simulink library "tpm"  (R2021b)
settings: Solver=VariableStepAuto  StartTime=0.0  StopTime=10.0  RelTol=1e-3
undefined symbols (not defined in the file or in its folder): ENUM_AN_LF, ENUM_AN_LR, ENUM_AN_RF, ENUM_AN_RR, ENUM_POWERSTA_OFF, ENUM_POWERSTA_OFFA, ENUM_POWERSTA_OFFC, ENUM_POWERSTA_ON, ENUM_POWERSTA_READY, ENUM_POWERSTA_STANDBY, ENUM_PWRSTASW_OFF, ENUM_PWRSTASW_OFFA, ENUM_PWRSTASW_OFFCHVCHRG, ENUM_PWRSTASW_STANDBY, KTPM_Delay_raw8, KTPM_WhlRotDir_enum_ovrdflg, KTPM_WhlRotDir_enum_ovrdval, TRUE, ZERO_FLOAT, ZERO_INT
libraries: simulink x58, hcu_lib x25, $bdroot x18
(part 6 of 8)

== system tpm/TPM/TPMS/TPMS/Learn/AutoLocation/IDIdentify/unlearnsensorfail  ==
  VTPM_ALLFIN_flg : Inport
  VINP_VehSpeed_kph : Inport  Port=2
  VTPM_IDLOCK_flg : Inport  Port=3
  GS1 : Inport  Port=4
  GS2 : Inport  Port=5
  GS3 : Inport  Port=6
  GS4 : Inport  Port=7
  VINP_TPMSResButt_flg : Inport  Port=8
  VINP_FlashunlearnSfali_flg : Inport  Port=9
  VINP_ChkStorge_flg : Inport  Port=10
  VINP_TPMSStorge_flg : Inport  Port=11
  Chart : Stateflow chart  TreatAsAtomicUnit=on
      settings: PortSchema="{\"entries\":[{\"content\":{\"sides\":[{\"content\":{\"connectorIds\":[\"In1\",\"In2\",\"In3\",\"In7\",\"In4\",\"In5\",\"In6\",\"In8\",\"In9\",\"In10\",\"In11\"]},\"type\":\"ConnectorPlacement.EquallySpacedRectSide\",\"uuid\":\"6d6ad79b-53cb-4fcc-b2ed-afc1b708014e\"},{\"content\":{\"connectorIds\":[\"Out1\",\"Out2\"],\"side\":\"RIGHT\"},\"type\":\"ConnectorPlacement.EquallySpacedRectSide\",\"uuid\":\"e1142f2b-ba58-4cb3-ba57-f7dfdeb40e8a\"},{\"content\":{\"connectorIds\":[],\"side\":\"TOP\"},\"type\":\"ConnectorPlacement.EquallySpacedRectSide\",\"uuid\":\"d6c2cba7-0cc1-4e16-8027-e1abdfd1a8ea\"}]},\"type\":\"ConnectorPlacement.EquallySpacedConnector\",\"uuid\":\"635c654b-7cdc-40ae-8580-2307d04d13e7\"}],\"packageUris\":[\"http://schema.mathworks.com/mf0/Connector/R2020b\"],\"version\":\"1.0\"}"
  Detect Increase4 : simulink/Logic and Bit Operations/Detect Increase  vinit=0.0  OutDataTypeStr=boolean
  SR_Latch : hcu_lib/Basic_Blocks/SR_Latch
  VTPM_unlearnSfali_flg : Outport
  VTPM_unlearnSfailvalid_enum : Outport  Port=2
  VTPM_unlockpopup_flg : Outport  Port=3
  wires:
  Chart/1(VTPM_unlearnSfali_flg) -> VTPM_unlearnSfali_flg/1, [VTPM_unlearnSfali_flg]
  GS1/1 -> Chart/7(VTPM_GS1_flg)
  GS4/1 -> Chart/6(VTPM_GS4_flg)
  GS3/1 -> Chart/5(VTPM_GS3_flg)
  GS2/1 -> Chart/4(VTPM_GS2_flg)
  VTPM_IDLOCK_flg/1 -> Chart/3(VTPM_IDLOCK_flg)
  VINP_VehSpeed_kph/1 -> Chart/2(VINP_VehSpeed_kph)
  VTPM_ALLFIN_flg/1 -> Chart/1(VTPM_ALLFIN_flg)
  VINP_FlashunlearnSfali_flg/1 -> Chart/9(VINP_FlashunlearnSfali_flg)
  VINP_ChkStorge_flg/1 -> Chart/10(VINP_ChkStorge_flg)
  VINP_TPMSStorge_flg/1 -> Chart/11(VINP_TPMSStorge_flg)
  SR_Latch/1 -> VTPM_unlearnSfailvalid_enum/1
  Detect Increase4/1 -> SR_Latch/1
  [VTPM_unlearnSfali_flg] -> Detect Increase4/1
  VINP_TPMSResButt_flg/1 -> [VINP_TPMSResButt_flg]
  [VINP_TPMSResButt_flg] -> Chart/8(VINP_TPMSResButt_flg)
  [VINP_TPMSResButt_flg] -> SR_Latch/2
  Chart/2(VTPM_unlockpopup_flg) -> VTPM_unlockpopup_flg/1

== system tpm/TPM/TPMS/TPMS/Learn/AutoLocation/WheelPosition/Subsystem ==
  VTPM_LFWpos_raw : Inport
  Constant : Constant  Value=KTPM_Delay_raw8
  If : If  IfExpression=u1 == 1  ElseIfExpressions=u1 ==2,u1 ==3,u1 ==4,u1 == 5,u1 ==6,u1 ==7,u1 ==8
  Merge1 : Merge  Inputs=9
  delay0 : Subsystem  TreatAsAtomicUnit=on
  delay1 : Subsystem  TreatAsAtomicUnit=on
  delay2 : Subsystem  TreatAsAtomicUnit=on
  delay3 : Subsystem  TreatAsAtomicUnit=on
  delay4 : Subsystem  TreatAsAtomicUnit=on
  delay5 : Subsystem  TreatAsAtomicUnit=on
  delay6 : Subsystem  TreatAsAtomicUnit=on
  delay7 : Subsystem  TreatAsAtomicUnit=on
  delay8 : Subsystem  TreatAsAtomicUnit=on
  VTPM_LFWP_raw16 : Outport
  wires:
  [VTPM_LFWP_raw16] -> delay3/1(In1)
  [VTPM_LFWP_raw16] -> delay1/1(In1)
  Constant/1 -> If/1
  Merge1/1 -> VTPM_LFWP_raw16/1
  [VTPM_LFWP_raw16] -> delay6/1(In1)
  [VTPM_LFWP_raw16] -> delay5/1(In1)
  [VTPM_LFWP_raw16] -> delay2/1(In1)
  [VTPM_LFWP_raw16] -> delay4/1(In1)
  [VTPM_LFWP_raw16] -> delay0/1(In1)
  VTPM_LFWpos_raw/1 -> [VTPM_LFWP_raw16]
  If/1 -> delay1/Action
  If/2 -> delay2/Action
  If/3 -> delay3/Action
  If/4 -> delay4/Action
  If/5 -> delay5/Action
  If/6 -> delay6/Action
  If/9 -> delay0/Action
  delay5/1(Out1) -> Merge1/5
  delay4/1(Out1) -> Merge1/4
  delay1/1(Out1) -> Merge1/1
  delay3/1(Out1) -> Merge1/3
  delay6/1(Out1) -> Merge1/6
  delay2/1(Out1) -> Merge1/2
  If/7 -> delay7/Action
  [VTPM_LFWP_raw16] -> delay7/1(In1)
  [VTPM_LFWP_raw16] -> delay8/1(In1)
  If/8 -> delay8/Action
  delay7/1(Out1) -> Merge1/7
  delay8/1(Out1) -> Merge1/8
  delay0/1(Out1) -> Merge1/9

== system tpm/TPM/TPMS/TPMS/Learn/AutoLocation/WheelPosition/Subsystem1 ==
  VTPM_RFWpos_raw : Inport
  Constant : Constant  Value=KTPM_Delay_raw8
  If : If  IfExpression=u1 == 1  ElseIfExpressions=u1 ==2,u1 ==3,u1 ==4,u1 == 5,u1 ==6,u1 ==7,u1 ==8
  Merge1 : Merge  Inputs=9
  delay0 : $bdroot/TPM/TPMS/TPMS/Learn/AutoLocation/WheelPosition/Subsystem/delay0  SystemSampleTime=-1  VariantActivationTime=update diagram  Latency=0  AutoFrameSizeCalculation=off
  delay1 : $bdroot/TPM/TPMS/TPMS/Learn/AutoLocation/WheelPosition/Subsystem/delay1  SystemSampleTime=-1  VariantActivationTime=update diagram  Latency=0  AutoFrameSizeCalculation=off
  delay2 : $bdroot/TPM/TPMS/TPMS/Learn/AutoLocation/WheelPosition/Subsystem/delay2  SystemSampleTime=-1  VariantActivationTime=update diagram  Latency=0  AutoFrameSizeCalculation=off
  delay3 : $bdroot/TPM/TPMS/TPMS/Learn/AutoLocation/WheelPosition/Subsystem/delay3  SystemSampleTime=-1  VariantActivationTime=update diagram  Latency=0  AutoFrameSizeCalculation=off
  delay4 : $bdroot/TPM/TPMS/TPMS/Learn/AutoLocation/WheelPosition/Subsystem/delay4  SystemSampleTime=-1  VariantActivationTime=update diagram  Latency=0  AutoFrameSizeCalculation=off
  delay5 : $bdroot/TPM/TPMS/TPMS/Learn/AutoLocation/WheelPosition/Subsystem/delay5  SystemSampleTime=-1  VariantActivationTime=update diagram  Latency=0  AutoFrameSizeCalculation=off
  delay6 : $bdroot/TPM/TPMS/TPMS/Learn/AutoLocation/WheelPosition/Subsystem/delay6  SystemSampleTime=-1  VariantActivationTime=update diagram  Latency=0  AutoFrameSizeCalculation=off
  delay7 : $bdroot/TPM/TPMS/TPMS/Learn/AutoLocation/WheelPosition/Subsystem/delay7  SystemSampleTime=-1  VariantActivationTime=update diagram  Latency=0  AutoFrameSizeCalculation=off
  delay8 : $bdroot/TPM/TPMS/TPMS/Learn/AutoLocation/WheelPosition/Subsystem/delay8  SystemSampleTime=-1  VariantActivationTime=update diagram  Latency=0  AutoFrameSizeCalculation=off
  VTPM_RFWP_raw16 : Outport
  wires:
  Merge1/1 -> VTPM_RFWP_raw16/1
  VTPM_RFWpos_raw/1 -> [VTPM_RFWP_raw16]
  [VTPM_RFWP_raw16] -> delay7/1
  delay7/1 -> Merge1/7
  delay8/1 -> Merge1/8
  delay0/1 -> Merge1/9
  [VTPM_RFWP_raw16] -> delay8/1
  [VTPM_RFWP_raw16] -> delay3/1
  If/2 -> delay2/Action
  [VTPM_RFWP_raw16] -> delay2/1
  [VTPM_RFWP_raw16] -> delay4/1
  If/1 -> delay1/Action
  [VTPM_RFWP_raw16] -> delay1/1
  If/9 -> delay0/Action
  If/3 -> delay3/Action
  [VTPM_RFWP_raw16] -> delay0/1
  delay2/1 -> Merge1/2
  delay5/1 -> Merge1/5
  [VTPM_RFWP_raw16] -> delay5/1
  delay6/1 -> Merge1/6
  If/6 -> delay6/Action
  If/8 -> delay8/Action
  delay3/1 -> Merge1/3
  If/5 -> delay5/Action
  [VTPM_RFWP_raw16] -> delay6/1
  If/4 -> delay4/Action
  delay4/1 -> Merge1/4
  delay1/1 -> Merge1/1
  If/7 -> delay7/Action
  Constant/1 -> If/1

== system tpm/TPM/TPMS/TPMS/Learn/AutoLocation/WheelPosition/Subsystem2 ==
  VTPM_LRWpos_raw : Inport
  Constant : Constant  Value=KTPM_Delay_raw8
  If : If  IfExpression=u1 == 1  ElseIfExpressions=u1 ==2,u1 ==3,u1 ==4,u1 == 5,u1 ==6,u1 ==7,u1 ==8
  Merge1 : Merge  Inputs=9
  delay0 : $bdroot/TPM/TPMS/TPMS/Learn/AutoLocation/WheelPosition/Subsystem/delay0  SystemSampleTime=-1  VariantActivationTime=update diagram  Latency=0  AutoFrameSizeCalculation=off
  delay1 : $bdroot/TPM/TPMS/TPMS/Learn/AutoLocation/WheelPosition/Subsystem/delay1  SystemSampleTime=-1  VariantActivationTime=update diagram  Latency=0  AutoFrameSizeCalculation=off
  delay2 : $bdroot/TPM/TPMS/TPMS/Learn/AutoLocation/WheelPosition/Subsystem/delay2  SystemSampleTime=-1  VariantActivationTime=update diagram  Latency=0  AutoFrameSizeCalculation=off
  delay3 : $bdroot/TPM/TPMS/TPMS/Learn/AutoLocation/WheelPosition/Subsystem/delay3  SystemSampleTime=-1  VariantActivationTime=update diagram  Latency=0  AutoFrameSizeCalculation=off
  delay4 : $bdroot/TPM/TPMS/TPMS/Learn/AutoLocation/WheelPosition/Subsystem/delay4  SystemSampleTime=-1  VariantActivationTime=update diagram  Latency=0  AutoFrameSizeCalculation=off
  delay5 : $bdroot/TPM/TPMS/TPMS/Learn/AutoLocation/WheelPosition/Subsystem/delay5  SystemSampleTime=-1  VariantActivationTime=update diagram  Latency=0  AutoFrameSizeCalculation=off
  delay6 : $bdroot/TPM/TPMS/TPMS/Learn/AutoLocation/WheelPosition/Subsystem/delay6  SystemSampleTime=-1  VariantActivationTime=update diagram  Latency=0  AutoFrameSizeCalculation=off
  delay7 : $bdroot/TPM/TPMS/TPMS/Learn/AutoLocation/WheelPosition/Subsystem/delay7  SystemSampleTime=-1  VariantActivationTime=update diagram  Latency=0  AutoFrameSizeCalculation=off
  delay8 : $bdroot/TPM/TPMS/TPMS/Learn/AutoLocation/WheelPosition/Subsystem/delay8  SystemSampleTime=-1  VariantActivationTime=update diagram  Latency=0  AutoFrameSizeCalculation=off
  VTPM_LRWP_raw16 : Outport
  wires:
  VTPM_LRWpos_raw/1 -> [VTPM_LRWP_raw16]
  Constant/1 -> If/1
  [VTPM_LRWP_raw16] -> delay5/1
  delay6/1 -> Merge1/6
  If/7 -> delay7/Action
  delay1/1 -> Merge1/1
  delay4/1 -> Merge1/4
  If/4 -> delay4/Action
  If/5 -> delay5/Action
  delay3/1 -> Merge1/3
  delay5/1 -> Merge1/5
  If/6 -> delay6/Action
  [VTPM_LRWP_raw16] -> delay0/1
  If/3 -> delay3/Action
  [VTPM_LRWP_raw16] -> delay3/1
  If/9 -> delay0/Action
  [VTPM_LRWP_raw16] -> delay8/1
  [VTPM_LRWP_raw16] -> delay2/1
  If/2 -> delay2/Action
  If/1 -> delay1/Action
  [VTPM_LRWP_raw16] -> delay1/1
  [VTPM_LRWP_raw16] -> delay4/1
  delay2/1 -> Merge1/2
  delay0/1 -> Merge1/9
  [VTPM_LRWP_raw16] -> delay7/1
  delay7/1 -> Merge1/7
  If/8 -> delay8/Action
  delay8/1 -> Merge1/8
  [VTPM_LRWP_raw16] -> delay6/1
  Merge1/1 -> VTPM_LRWP_raw16/1

== system tpm/TPM/TPMS/TPMS/Learn/AutoLocation/WheelPosition/Subsystem3 ==
  VTPM_RRWpos_raw : Inport
  Constant : Constant  Value=KTPM_Delay_raw8
  If : If  IfExpression=u1 == 1  ElseIfExpressions=u1 ==2,u1 ==3,u1 ==4,u1 == 5,u1 ==6,u1 ==7,u1 ==8
  Merge1 : Merge  Inputs=9
  delay0 : Subsystem  TreatAsAtomicUnit=on
  delay1 : Subsystem  TreatAsAtomicUnit=on
  delay2 : Subsystem  TreatAsAtomicUnit=on
  delay3 : Subsystem  TreatAsAtomicUnit=on
  delay4 : Subsystem  TreatAsAtomicUnit=on
  delay5 : Subsystem  TreatAsAtomicUnit=on
  delay6 : Subsystem  TreatAsAtomicUnit=on
  delay7 : Subsystem  TreatAsAtomicUnit=on
  delay8 : Subsystem  TreatAsAtomicUnit=on
  VTPM_RRWP_raw16 : Outport
  wires:
  Merge1/1 -> VTPM_RRWP_raw16/1
  [VTPM_RRWP_raw16] -> delay6/1(In1)
  delay8/1(Out1) -> Merge1/8
  If/8 -> delay8/Action
  delay7/1(Out1) -> Merge1/7
  [VTPM_RRWP_raw16] -> delay7/1(In1)
  delay0/1(Out1) -> Merge1/9
  delay2/1(Out1) -> Merge1/2
  [VTPM_RRWP_raw16] -> delay4/1(In1)
  [VTPM_RRWP_raw16] -> delay1/1(In1)
  If/1 -> delay1/Action
  If/2 -> delay2/Action
  [VTPM_RRWP_raw16] -> delay2/1(In1)
  [VTPM_RRWP_raw16] -> delay8/1(In1)
  If/9 -> delay0/Action
  [VTPM_RRWP_raw16] -> delay3/1(In1)
  If/3 -> delay3/Action
  [VTPM_RRWP_raw16] -> delay0/1(In1)
  If/6 -> delay6/Action
  delay5/1(Out1) -> Merge1/5
  delay3/1(Out1) -> Merge1/3
  If/5 -> delay5/Action
  If/4 -> delay4/Action
  delay4/1(Out1) -> Merge1/4
  delay1/1(Out1) -> Merge1/1
  If/7 -> delay7/Action
  delay6/1(Out1) -> Merge1/6
  [VTPM_RRWP_raw16] -> delay5/1(In1)
  Constant/1 -> If/1
  VTPM_RRWpos_raw/1 -> [VTPM_RRWP_raw16]

== system tpm/TPM/TPMS/TPMS/Learn/AutoLocation/IDIdentify/Subsystem1/Enabled Subsystem1 ==
  C : Inport
  LFM1 : Inport  Port=2
  Enable : EnablePort
  Data Type Conversion{1..8} (8 alike) : DataTypeConversion  OutDataTypeStr=int16
  Data Type Conversion9 : DataTypeConversion  OutDataTypeStr=uint8
  MATLAB Function : MATLAB Function  TreatAsAtomicUnit=on
  Unit Delay{1..8} (8 alike) : UnitDelay  SampleTime=-1  HasFrameUpgradeWarning=on
  S : Outport
  wires:
  Data Type Conversion9/1 -> S/1
  Data Type Conversion3/1 -> [X4]
  Data Type Conversion2/1 -> [X3]
  Data Type Conversion1/1 -> [X2]
  LFM1/1 -> MATLAB Function/2(Min)
  MATLAB Function/1(S) -> Data Type Conversion9/1
  C/1 -> MATLAB Function/1(C)
  MATLAB Function/2(Y2) -> Unit Delay1/1
  MATLAB Function/3(Y3) -> Unit Delay2/1
  MATLAB Function/4(Y4) -> Unit Delay3/1
  Unit Delay1/1 -> Data Type Conversion1/1
  Unit Delay2/1 -> Data Type Conversion2/1
  Unit Delay3/1 -> Data Type Conversion3/1
  [X2] -> MATLAB Function/3(X2)
  [X3] -> MATLAB Function/4(X3)
  [X4] -> MATLAB Function/5(X4)
  Unit Delay6/1 -> Data Type Conversion5/1
  Unit Delay5/1 -> Data Type Conversion4/1
  MATLAB Function/6(Y6) -> Unit Delay6/1
  MATLAB Function/5(Y5) -> Unit Delay5/1
  Data Type Conversion4/1 -> [X5]
  Data Type Conversion5/1 -> [X6]
  [X5] -> MATLAB Function/6(X5)
  [X6] -> MATLAB Function/7(X6)
  [X7] -> MATLAB Function/8(X7)
  [X8] -> MATLAB Function/9(X8)
  Data Type Conversion6/1 -> [X7]
  MATLAB Function/7(Y7) -> Unit Delay4/1
  Unit Delay4/1 -> Data Type Conversion6/1
  Unit Delay7/1 -> Data Type Conversion7/1
  Data Type Conversion7/1 -> [X8]
  MATLAB Function/8(Y8) -> Unit Delay7/1
  MATLAB Function/9(Y9) -> Unit Delay8/1
  Data Type Conversion8/1 -> [X9]
  Unit Delay8/1 -> Data Type Conversion8/1
  [X9] -> MATLAB Function/10(X9)

== system tpm/TPM/TPMS/TPMS/Learn/AutoLocation/IDIdentify/Subsystem1/Enabled Subsystem2 ==
  C : Inport
  LFM1 : Inport  Port=2
  Enable : EnablePort
  Data Type Conversion{1..8} (8 alike) : DataTypeConversion  OutDataTypeStr=int16
  Data Type Conversion9 : DataTypeConversion  OutDataTypeStr=uint8
  MATLAB Function : MATLAB Function  TreatAsAtomicUnit=on
  Unit Delay{1..8} (8 alike) : UnitDelay  SampleTime=-1  HasFrameUpgradeWarning=on
  S : Outport
  wires:
  Data Type Conversion9/1 -> S/1
  [X9] -> MATLAB Function/10(X9)
  Unit Delay8/1 -> Data Type Conversion8/1
  Data Type Conversion8/1 -> [X9]
  MATLAB Function/9(Y9) -> Unit Delay8/1
  MATLAB Function/8(Y8) -> Unit Delay7/1
  Data Type Conversion7/1 -> [X8]
  Unit Delay7/1 -> Data Type Conversion7/1
  Unit Delay4/1 -> Data Type Conversion6/1
  MATLAB Function/7(Y7) -> Unit Delay4/1
  Data Type Conversion6/1 -> [X7]
  [X8] -> MATLAB Function/9(X8)
  [X7] -> MATLAB Function/8(X7)
  [X6] -> MATLAB Function/7(X6)
  [X5] -> MATLAB Function/6(X5)
  Data Type Conversion5/1 -> [X6]
  Data Type Conversion4/1 -> [X5]
  MATLAB Function/5(Y5) -> Unit Delay5/1
  MATLAB Function/6(Y6) -> Unit Delay6/1
  Unit Delay5/1 -> Data Type Conversion4/1
  Unit Delay6/1 -> Data Type Conversion5/1
  [X4] -> MATLAB Function/5(X4)
  [X3] -> MATLAB Function/4(X3)
  [X2] -> MATLAB Function/3(X2)
  Unit Delay3/1 -> Data Type Conversion3/1
  Unit Delay2/1 -> Data Type Conversion2/1
  Unit Delay1/1 -> Data Type Conversion1/1
  MATLAB Function/4(Y4) -> Unit Delay3/1
  MATLAB Function/3(Y3) -> Unit Delay2/1
  MATLAB Function/2(Y2) -> Unit Delay1/1
  C/1 -> MATLAB Function/1(C)
  MATLAB Function/1(S) -> Data Type Conversion9/1
  LFM1/1 -> MATLAB Function/2(Min)
  Data Type Conversion1/1 -> [X2]
  Data Type Conversion2/1 -> [X3]
  Data Type Conversion3/1 -> [X4]

== system tpm/TPM/TPMS/TPMS/Learn/AutoLocation/IDIdentify/Subsystem1/Enabled Subsystem3 ==
  C : Inport
  LFM1 : Inport  Port=2
  Enable : EnablePort
  Data Type Conversion{1..8} (8 alike) : DataTypeConversion  OutDataTypeStr=int16
  Data Type Conversion9 : DataTypeConversion  OutDataTypeStr=uint8
  MATLAB Function : MATLAB Function  TreatAsAtomicUnit=on
  Unit Delay{1..8} (8 alike) : UnitDelay  SampleTime=-1  HasFrameUpgradeWarning=on
  S : Outport
  wires:
  Data Type Conversion9/1 -> S/1
  Data Type Conversion3/1 -> [X4]
  Data Type Conversion2/1 -> [X3]
  Data Type Conversion1/1 -> [X2]
  LFM1/1 -> MATLAB Function/2(Min)
  MATLAB Function/1(S) -> Data Type Conversion9/1
  C/1 -> MATLAB Function/1(C)
  MATLAB Function/2(Y2) -> Unit Delay1/1
  MATLAB Function/3(Y3) -> Unit Delay2/1
  MATLAB Function/4(Y4) -> Unit Delay3/1
  Unit Delay1/1 -> Data Type Conversion1/1
  Unit Delay2/1 -> Data Type Conversion2/1
  Unit Delay3/1 -> Data Type Conversion3/1
  [X2] -> MATLAB Function/3(X2)
  [X3] -> MATLAB Function/4(X3)
  [X4] -> MATLAB Function/5(X4)
  Unit Delay6/1 -> Data Type Conversion5/1
  Unit Delay5/1 -> Data Type Conversion4/1
  MATLAB Function/6(Y6) -> Unit Delay6/1
  MATLAB Function/5(Y5) -> Unit Delay5/1
  Data Type Conversion4/1 -> [X5]
  Data Type Conversion5/1 -> [X6]
  [X5] -> MATLAB Function/6(X5)
  [X6] -> MATLAB Function/7(X6)
  [X7] -> MATLAB Function/8(X7)
  [X8] -> MATLAB Function/9(X8)
  Data Type Conversion6/1 -> [X7]
  MATLAB Function/7(Y7) -> Unit Delay4/1
  Unit Delay4/1 -> Data Type Conversion6/1
  Unit Delay7/1 -> Data Type Conversion7/1
  Data Type Conversion7/1 -> [X8]
  MATLAB Function/8(Y8) -> Unit Delay7/1
  MATLAB Function/9(Y9) -> Unit Delay8/1
  Data Type Conversion8/1 -> [X9]
  Unit Delay8/1 -> Data Type Conversion8/1
  [X9] -> MATLAB Function/10(X9)

== system tpm/TPM/TPMS/TPMS/Learn/AutoLocation/IDIdentify/Subsystem1/Enabled Subsystem5 ==
  C : Inport
  LFM1 : Inport  Port=2
  Enable : EnablePort
  Data Type Conversion{1..8} (8 alike) : DataTypeConversion  OutDataTypeStr=int16
  Data Type Conversion9 : DataTypeConversion  OutDataTypeStr=uint8
  MATLAB Function : MATLAB Function  TreatAsAtomicUnit=on
  Unit Delay{1..8} (8 alike) : UnitDelay  SampleTime=-1  HasFrameUpgradeWarning=on
  S : Outport
  wires:
  Data Type Conversion9/1 -> S/1
  [X9] -> MATLAB Function/10(X9)
  Unit Delay8/1 -> Data Type Conversion8/1
  Data Type Conversion8/1 -> [X9]
  MATLAB Function/9(Y9) -> Unit Delay8/1
  MATLAB Function/8(Y8) -> Unit Delay7/1
  Data Type Conversion7/1 -> [X8]
  Unit Delay7/1 -> Data Type Conversion7/1
  Unit Delay4/1 -> Data Type Conversion6/1
  MATLAB Function/7(Y7) -> Unit Delay4/1
  Data Type Conversion6/1 -> [X7]
  [X8] -> MATLAB Function/9(X8)
  [X7] -> MATLAB Function/8(X7)
  [X6] -> MATLAB Function/7(X6)
  [X5] -> MATLAB Function/6(X5)
  Data Type Conversion5/1 -> [X6]
  Data Type Conversion4/1 -> [X5]
  MATLAB Function/5(Y5) -> Unit Delay5/1
  MATLAB Function/6(Y6) -> Unit Delay6/1
  Unit Delay5/1 -> Data Type Conversion4/1
  Unit Delay6/1 -> Data Type Conversion5/1
  [X4] -> MATLAB Function/5(X4)
  [X3] -> MATLAB Function/4(X3)
  [X2] -> MATLAB Function/3(X2)
  Unit Delay3/1 -> Data Type Conversion3/1
  Unit Delay2/1 -> Data Type Conversion2/1
  Unit Delay1/1 -> Data Type Conversion1/1
  MATLAB Function/4(Y4) -> Unit Delay3/1
  MATLAB Function/3(Y3) -> Unit Delay2/1
  MATLAB Function/2(Y2) -> Unit Delay1/1
  C/1 -> MATLAB Function/1(C)
  MATLAB Function/1(S) -> Data Type Conversion9/1
  LFM1/1 -> MATLAB Function/2(Min)
  Data Type Conversion1/1 -> [X2]
  Data Type Conversion2/1 -> [X3]
  Data Type Conversion3/1 -> [X4]

== system tpm/TPM/TPMS/TPMS/Learn/AutoLocation/IDIdentify/Subsystem2/Enabled Subsystem1 ==
  C : Inport
  LFM1 : Inport  Port=2
  Enable : EnablePort
  Data Type Conversion{1..8} (8 alike) : DataTypeConversion  OutDataTypeStr=int16
  Data Type Conversion9 : DataTypeConversion  OutDataTypeStr=uint8
  MATLAB Function : MATLAB Function  TreatAsAtomicUnit=on
  Unit Delay{1..8} (8 alike) : UnitDelay  SampleTime=-1  HasFrameUpgradeWarning=on
  S : Outport
  wires:
  [X9] -> MATLAB Function/10(X9)
  Unit Delay8/1 -> Data Type Conversion8/1
  Data Type Conversion8/1 -> [X9]
  MATLAB Function/9(Y9) -> Unit Delay8/1
  MATLAB Function/8(Y8) -> Unit Delay7/1
  Data Type Conversion7/1 -> [X8]
  Unit Delay7/1 -> Data Type Conversion7/1
  Unit Delay4/1 -> Data Type Conversion6/1
  MATLAB Function/7(Y7) -> Unit Delay4/1
  Data Type Conversion6/1 -> [X7]
  [X8] -> MATLAB Function/9(X8)
  [X7] -> MATLAB Function/8(X7)
  [X6] -> MATLAB Function/7(X6)
  [X5] -> MATLAB Function/6(X5)
  Data Type Conversion5/1 -> [X6]
  Data Type Conversion4/1 -> [X5]
  MATLAB Function/5(Y5) -> Unit Delay5/1
  MATLAB Function/6(Y6) -> Unit Delay6/1
  Unit Delay5/1 -> Data Type Conversion4/1
  Unit Delay6/1 -> Data Type Conversion5/1
  [X4] -> MATLAB Function/5(X4)
  [X3] -> MATLAB Function/4(X3)
  [X2] -> MATLAB Function/3(X2)
  Unit Delay3/1 -> Data Type Conversion3/1
  Unit Delay2/1 -> Data Type Conversion2/1
  Unit Delay1/1 -> Data Type Conversion1/1
  MATLAB Function/4(Y4) -> Unit Delay3/1
  MATLAB Function/3(Y3) -> Unit Delay2/1
  MATLAB Function/2(Y2) -> Unit Delay1/1
  C/1 -> MATLAB Function/1(C)
  MATLAB Function/1(S) -> Data Type Conversion9/1
  LFM1/1 -> MATLAB Function/2(Min)
  Data Type Conversion1/1 -> [X2]
  Data Type Conversion2/1 -> [X3]
  Data Type Conversion3/1 -> [X4]
  Data Type Conversion9/1 -> S/1

== system tpm/TPM/TPMS/TPMS/Learn/AutoLocation/IDIdentify/Subsystem2/Enabled Subsystem2 ==
  C : Inport
  LFM1 : Inport  Port=2
  Enable : EnablePort
  Data Type Conversion{1..8} (8 alike) : DataTypeConversion  OutDataTypeStr=int16
  Data Type Conversion9 : DataTypeConversion  OutDataTypeStr=uint8
  MATLAB Function : MATLAB Function  TreatAsAtomicUnit=on
  Unit Delay{1..8} (8 alike) : UnitDelay  SampleTime=-1  HasFrameUpgradeWarning=on
  S : Outport
  wires:
  Data Type Conversion3/1 -> [X4]
  Data Type Conversion2/1 -> [X3]
  Data Type Conversion1/1 -> [X2]
  LFM1/1 -> MATLAB Function/2(Min)
  MATLAB Function/1(S) -> Data Type Conversion9/1
  C/1 -> MATLAB Function/1(C)
  MATLAB Function/2(Y2) -> Unit Delay1/1
  MATLAB Function/3(Y3) -> Unit Delay2/1
  MATLAB Function/4(Y4) -> Unit Delay3/1
  Unit Delay1/1 -> Data Type Conversion1/1
  Unit Delay2/1 -> Data Type Conversion2/1
  Unit Delay3/1 -> Data Type Conversion3/1
  [X2] -> MATLAB Function/3(X2)
  [X3] -> MATLAB Function/4(X3)
  [X4] -> MATLAB Function/5(X4)
  Unit Delay6/1 -> Data Type Conversion5/1
  Unit Delay5/1 -> Data Type Conversion4/1
  MATLAB Function/6(Y6) -> Unit Delay6/1
  MATLAB Function/5(Y5) -> Unit Delay5/1
  Data Type Conversion4/1 -> [X5]
  Data Type Conversion5/1 -> [X6]
  [X5] -> MATLAB Function/6(X5)
  [X6] -> MATLAB Function/7(X6)
  [X7] -> MATLAB Function/8(X7)
  [X8] -> MATLAB Function/9(X8)
  Data Type Conversion6/1 -> [X7]
  MATLAB Function/7(Y7) -> Unit Delay4/1
  Unit Delay4/1 -> Data Type Conversion6/1
  Unit Delay7/1 -> Data Type Conversion7/1
  Data Type Conversion7/1 -> [X8]
  MATLAB Function/8(Y8) -> Unit Delay7/1
  MATLAB Function/9(Y9) -> Unit Delay8/1
  Data Type Conversion8/1 -> [X9]
  Unit Delay8/1 -> Data Type Conversion8/1
  [X9] -> MATLAB Function/10(X9)
  Data Type Conversion9/1 -> S/1

== system tpm/TPM/TPMS/TPMS/Learn/AutoLocation/IDIdentify/Subsystem2/Enabled Subsystem3 ==
  C : Inport
  LFM1 : Inport  Port=2
  Enable : EnablePort
  Data Type Conversion{1..8} (8 alike) : DataTypeConversion  OutDataTypeStr=int16
  Data Type Conversion9 : DataTypeConversion  OutDataTypeStr=uint8
  MATLAB Function : MATLAB Function  TreatAsAtomicUnit=on
  Unit Delay{1..8} (8 alike) : UnitDelay  SampleTime=-1  HasFrameUpgradeWarning=on
  S : Outport
  wires:
  [X9] -> MATLAB Function/10(X9)
  Unit Delay8/1 -> Data Type Conversion8/1
  Data Type Conversion8/1 -> [X9]
  MATLAB Function/9(Y9) -> Unit Delay8/1
  MATLAB Function/8(Y8) -> Unit Delay7/1
  Data Type Conversion7/1 -> [X8]
  Unit Delay7/1 -> Data Type Conversion7/1
  Unit Delay4/1 -> Data Type Conversion6/1
  MATLAB Function/7(Y7) -> Unit Delay4/1
  Data Type Conversion6/1 -> [X7]
  [X8] -> MATLAB Function/9(X8)
  [X7] -> MATLAB Function/8(X7)
  [X6] -> MATLAB Function/7(X6)
  [X5] -> MATLAB Function/6(X5)
  Data Type Conversion5/1 -> [X6]
  Data Type Conversion4/1 -> [X5]
  MATLAB Function/5(Y5) -> Unit Delay5/1
  MATLAB Function/6(Y6) -> Unit Delay6/1
  Unit Delay5/1 -> Data Type Conversion4/1
  Unit Delay6/1 -> Data Type Conversion5/1
  [X4] -> MATLAB Function/5(X4)
  [X3] -> MATLAB Function/4(X3)
  [X2] -> MATLAB Function/3(X2)
  Unit Delay3/1 -> Data Type Conversion3/1
  Unit Delay2/1 -> Data Type Conversion2/1
  Unit Delay1/1 -> Data Type Conversion1/1
  MATLAB Function/4(Y4) -> Unit Delay3/1
  MATLAB Function/3(Y3) -> Unit Delay2/1
  MATLAB Function/2(Y2) -> Unit Delay1/1
  C/1 -> MATLAB Function/1(C)
  MATLAB Function/1(S) -> Data Type Conversion9/1
  LFM1/1 -> MATLAB Function/2(Min)
  Data Type Conversion1/1 -> [X2]
  Data Type Conversion2/1 -> [X3]
  Data Type Conversion3/1 -> [X4]
  Data Type Conversion9/1 -> S/1

== system tpm/TPM/TPMS/TPMS/Learn/AutoLocation/IDIdentify/Subsystem2/Enabled Subsystem5 ==
  C : Inport
  LFM1 : Inport  Port=2
  Enable : EnablePort
  Data Type Conversion{1..8} (8 alike) : DataTypeConversion  OutDataTypeStr=int16
  Data Type Conversion9 : DataTypeConversion  OutDataTypeStr=uint8
  MATLAB Function : MATLAB Function  TreatAsAtomicUnit=on
  Unit Delay{1..8} (8 alike) : UnitDelay  SampleTime=-1  HasFrameUpgradeWarning=on
  S : Outport
  wires:
  Data Type Conversion3/1 -> [X4]
  Data Type Conversion2/1 -> [X3]
  Data Type Conversion1/1 -> [X2]
  LFM1/1 -> MATLAB Function/2(Min)
  MATLAB Function/1(S) -> Data Type Conversion9/1
  C/1 -> MATLAB Function/1(C)
  MATLAB Function/2(Y2) -> Unit Delay1/1
  MATLAB Function/3(Y3) -> Unit Delay2/1
  MATLAB Function/4(Y4) -> Unit Delay3/1
  Unit Delay1/1 -> Data Type Conversion1/1
  Unit Delay2/1 -> Data Type Conversion2/1
  Unit Delay3/1 -> Data Type Conversion3/1
  [X2] -> MATLAB Function/3(X2)
  [X3] -> MATLAB Function/4(X3)
  [X4] -> MATLAB Function/5(X4)
  Unit Delay6/1 -> Data Type Conversion5/1
  Unit Delay5/1 -> Data Type Conversion4/1
  MATLAB Function/6(Y6) -> Unit Delay6/1
  MATLAB Function/5(Y5) -> Unit Delay5/1
  Data Type Conversion4/1 -> [X5]
  Data Type Conversion5/1 -> [X6]
  [X5] -> MATLAB Function/6(X5)
  [X6] -> MATLAB Function/7(X6)
  [X7] -> MATLAB Function/8(X7)
  [X8] -> MATLAB Function/9(X8)
  Data Type Conversion6/1 -> [X7]
  MATLAB Function/7(Y7) -> Unit Delay4/1
  Unit Delay4/1 -> Data Type Conversion6/1
  Unit Delay7/1 -> Data Type Conversion7/1
  Data Type Conversion7/1 -> [X8]
  MATLAB Function/8(Y8) -> Unit Delay7/1
  MATLAB Function/9(Y9) -> Unit Delay8/1
  Data Type Conversion8/1 -> [X9]
  Unit Delay8/1 -> Data Type Conversion8/1
  [X9] -> MATLAB Function/10(X9)
  Data Type Conversion9/1 -> S/1

== system tpm/TPM/TPMS/TPMS/Learn/AutoLocation/IDIdentify/Subsystem3/Enabled Subsystem1 ==
  C : Inport
  LFM1 : Inport  Port=2
  Enable : EnablePort
  Data Type Conversion{1..8} (8 alike) : DataTypeConversion  OutDataTypeStr=int16
  Data Type Conversion9 : DataTypeConversion  OutDataTypeStr=uint8
  MATLAB Function : MATLAB Function  TreatAsAtomicUnit=on
  Unit Delay{1..8} (8 alike) : UnitDelay  SampleTime=-1  HasFrameUpgradeWarning=on
  S : Outport
  wires:
  Data Type Conversion9/1 -> S/1
  Data Type Conversion3/1 -> [X4]
  Data Type Conversion2/1 -> [X3]
  Data Type Conversion1/1 -> [X2]
  LFM1/1 -> MATLAB Function/2(Min)
  MATLAB Function/1(S) -> Data Type Conversion9/1
  C/1 -> MATLAB Function/1(C)
  MATLAB Function/2(Y2) -> Unit Delay1/1
  MATLAB Function/3(Y3) -> Unit Delay2/1
  MATLAB Function/4(Y4) -> Unit Delay3/1
  Unit Delay1/1 -> Data Type Conversion1/1
  Unit Delay2/1 -> Data Type Conversion2/1
  Unit Delay3/1 -> Data Type Conversion3/1
  [X2] -> MATLAB Function/3(X2)
  [X3] -> MATLAB Function/4(X3)
  [X4] -> MATLAB Function/5(X4)
  Unit Delay6/1 -> Data Type Conversion5/1
  Unit Delay5/1 -> Data Type Conversion4/1
  MATLAB Function/6(Y6) -> Unit Delay6/1
  MATLAB Function/5(Y5) -> Unit Delay5/1
  Data Type Conversion4/1 -> [X5]
  Data Type Conversion5/1 -> [X6]
  [X5] -> MATLAB Function/6(X5)
  [X6] -> MATLAB Function/7(X6)
  [X7] -> MATLAB Function/8(X7)
  [X8] -> MATLAB Function/9(X8)
  Data Type Conversion6/1 -> [X7]
  MATLAB Function/7(Y7) -> Unit Delay4/1
  Unit Delay4/1 -> Data Type Conversion6/1
  Unit Delay7/1 -> Data Type Conversion7/1
  Data Type Conversion7/1 -> [X8]
  MATLAB Function/8(Y8) -> Unit Delay7/1
  MATLAB Function/9(Y9) -> Unit Delay8/1
  Data Type Conversion8/1 -> [X9]
  Unit Delay8/1 -> Data Type Conversion8/1
  [X9] -> MATLAB Function/10(X9)

== system tpm/TPM/TPMS/TPMS/Learn/AutoLocation/IDIdentify/Subsystem3/Enabled Subsystem2 ==
  C : Inport
  LFM1 : Inport  Port=2
  Enable : EnablePort
  Data Type Conversion{1..8} (8 alike) : DataTypeConversion  OutDataTypeStr=int16
  Data Type Conversion9 : DataTypeConversion  OutDataTypeStr=uint8
  MATLAB Function : MATLAB Function  TreatAsAtomicUnit=on
  Unit Delay{1..8} (8 alike) : UnitDelay  SampleTime=-1  HasFrameUpgradeWarning=on
  S : Outport
  wires:
  Data Type Conversion9/1 -> S/1
  [X9] -> MATLAB Function/10(X9)
  Unit Delay8/1 -> Data Type Conversion8/1
  Data Type Conversion8/1 -> [X9]
  MATLAB Function/9(Y9) -> Unit Delay8/1
  MATLAB Function/8(Y8) -> Unit Delay7/1
  Data Type Conversion7/1 -> [X8]
  Unit Delay7/1 -> Data Type Conversion7/1
  Unit Delay4/1 -> Data Type Conversion6/1
  MATLAB Function/7(Y7) -> Unit Delay4/1
  Data Type Conversion6/1 -> [X7]
  [X8] -> MATLAB Function/9(X8)
  [X7] -> MATLAB Function/8(X7)
  [X6] -> MATLAB Function/7(X6)
  [X5] -> MATLAB Function/6(X5)
  Data Type Conversion5/1 -> [X6]
  Data Type Conversion4/1 -> [X5]
  MATLAB Function/5(Y5) -> Unit Delay5/1
  MATLAB Function/6(Y6) -> Unit Delay6/1
  Unit Delay5/1 -> Data Type Conversion4/1
  Unit Delay6/1 -> Data Type Conversion5/1
  [X4] -> MATLAB Function/5(X4)
  [X3] -> MATLAB Function/4(X3)
  [X2] -> MATLAB Function/3(X2)
  Unit Delay3/1 -> Data Type Conversion3/1
  Unit Delay2/1 -> Data Type Conversion2/1
  Unit Delay1/1 -> Data Type Conversion1/1
  MATLAB Function/4(Y4) -> Unit Delay3/1
  MATLAB Function/3(Y3) -> Unit Delay2/1
  MATLAB Function/2(Y2) -> Unit Delay1/1
  C/1 -> MATLAB Function/1(C)
  MATLAB Function/1(S) -> Data Type Conversion9/1
  LFM1/1 -> MATLAB Function/2(Min)
  Data Type Conversion1/1 -> [X2]
  Data Type Conversion2/1 -> [X3]
  Data Type Conversion3/1 -> [X4]

== system tpm/TPM/TPMS/TPMS/Learn/AutoLocation/IDIdentify/Subsystem3/Enabled Subsystem3 ==
  C : Inport
  LFM1 : Inport  Port=2
  Enable : EnablePort
  Data Type Conversion{1..8} (8 alike) : DataTypeConversion  OutDataTypeStr=int16
  Data Type Conversion9 : DataTypeConversion  OutDataTypeStr=uint8
  MATLAB Function : MATLAB Function  TreatAsAtomicUnit=on
  Unit Delay{1..8} (8 alike) : UnitDelay  SampleTime=-1  HasFrameUpgradeWarning=on
  S : Outport
  wires:
  Data Type Conversion9/1 -> S/1
  Data Type Conversion3/1 -> [X4]
  Data Type Conversion2/1 -> [X3]
  Data Type Conversion1/1 -> [X2]
  LFM1/1 -> MATLAB Function/2(Min)
  MATLAB Function/1(S) -> Data Type Conversion9/1
  C/1 -> MATLAB Function/1(C)
  MATLAB Function/2(Y2) -> Unit Delay1/1
  MATLAB Function/3(Y3) -> Unit Delay2/1
  MATLAB Function/4(Y4) -> Unit Delay3/1
  Unit Delay1/1 -> Data Type Conversion1/1
  Unit Delay2/1 -> Data Type Conversion2/1
  Unit Delay3/1 -> Data Type Conversion3/1
  [X2] -> MATLAB Function/3(X2)
  [X3] -> MATLAB Function/4(X3)
  [X4] -> MATLAB Function/5(X4)
  Unit Delay6/1 -> Data Type Conversion5/1
  Unit Delay5/1 -> Data Type Conversion4/1
  MATLAB Function/6(Y6) -> Unit Delay6/1
  MATLAB Function/5(Y5) -> Unit Delay5/1
  Data Type Conversion4/1 -> [X5]
  Data Type Conversion5/1 -> [X6]
  [X5] -> MATLAB Function/6(X5)
  [X6] -> MATLAB Function/7(X6)
  [X7] -> MATLAB Function/8(X7)
  [X8] -> MATLAB Function/9(X8)
  Data Type Conversion6/1 -> [X7]
  MATLAB Function/7(Y7) -> Unit Delay4/1
  Unit Delay4/1 -> Data Type Conversion6/1
  Unit Delay7/1 -> Data Type Conversion7/1
  Data Type Conversion7/1 -> [X8]
  MATLAB Function/8(Y8) -> Unit Delay7/1
  MATLAB Function/9(Y9) -> Unit Delay8/1
  Data Type Conversion8/1 -> [X9]
  Unit Delay8/1 -> Data Type Conversion8/1
  [X9] -> MATLAB Function/10(X9)

== system tpm/TPM/TPMS/TPMS/Learn/AutoLocation/IDIdentify/Subsystem3/Enabled Subsystem5 ==
  C : Inport
  LFM1 : Inport  Port=2
  Enable : EnablePort
  Data Type Conversion{1..8} (8 alike) : DataTypeConversion  OutDataTypeStr=int16
  Data Type Conversion9 : DataTypeConversion  OutDataTypeStr=uint8
  MATLAB Function : MATLAB Function  TreatAsAtomicUnit=on
  Unit Delay{1..8} (8 alike) : UnitDelay  SampleTime=-1  HasFrameUpgradeWarning=on
  S : Outport
  wires:
  Data Type Conversion9/1 -> S/1
  [X9] -> MATLAB Function/10(X9)
  Unit Delay8/1 -> Data Type Conversion8/1
  Data Type Conversion8/1 -> [X9]
  MATLAB Function/9(Y9) -> Unit Delay8/1
  MATLAB Function/8(Y8) -> Unit Delay7/1
  Data Type Conversion7/1 -> [X8]
  Unit Delay7/1 -> Data Type Conversion7/1
  Unit Delay4/1 -> Data Type Conversion6/1
  MATLAB Function/7(Y7) -> Unit Delay4/1
  Data Type Conversion6/1 -> [X7]
  [X8] -> MATLAB Function/9(X8)
  [X7] -> MATLAB Function/8(X7)
  [X6] -> MATLAB Function/7(X6)
  [X5] -> MATLAB Function/6(X5)
  Data Type Conversion5/1 -> [X6]
  Data Type Conversion4/1 -> [X5]
  MATLAB Function/5(Y5) -> Unit Delay5/1
  MATLAB Function/6(Y6) -> Unit Delay6/1
  Unit Delay5/1 -> Data Type Conversion4/1
  Unit Delay6/1 -> Data Type Conversion5/1
  [X4] -> MATLAB Function/5(X4)
  [X3] -> MATLAB Function/4(X3)
  [X2] -> MATLAB Function/3(X2)
  Unit Delay3/1 -> Data Type Conversion3/1
  Unit Delay2/1 -> Data Type Conversion2/1
  Unit Delay1/1 -> Data Type Conversion1/1
  MATLAB Function/4(Y4) -> Unit Delay3/1
  MATLAB Function/3(Y3) -> Unit Delay2/1
  MATLAB Function/2(Y2) -> Unit Delay1/1
  C/1 -> MATLAB Function/1(C)
  MATLAB Function/1(S) -> Data Type Conversion9/1
  LFM1/1 -> MATLAB Function/2(Min)
  Data Type Conversion1/1 -> [X2]
  Data Type Conversion2/1 -> [X3]
  Data Type Conversion3/1 -> [X4]

== system tpm/TPM/TPMS/TPMS/Learn/AutoLocation/IDIdentify/Subsystem7/Enabled Subsystem1 ==
  C : Inport
  LFM1 : Inport  Port=2
  Enable : EnablePort
  Data Type Conversion{1..8} (8 alike) : DataTypeConversion  OutDataTypeStr=int16
  Data Type Conversion9 : DataTypeConversion  OutDataTypeStr=uint8
  MATLAB Function : MATLAB Function  TreatAsAtomicUnit=on
  Unit Delay{1..8} (8 alike) : UnitDelay  SampleTime=-1  HasFrameUpgradeWarning=on
  S : Outport
  wires:
  [X9] -> MATLAB Function/10(X9)
  Unit Delay8/1 -> Data Type Conversion8/1
  Data Type Conversion8/1 -> [X9]
  MATLAB Function/9(Y9) -> Unit Delay8/1
  MATLAB Function/8(Y8) -> Unit Delay7/1
  Data Type Conversion7/1 -> [X8]
  Unit Delay7/1 -> Data Type Conversion7/1
  Unit Delay4/1 -> Data Type Conversion6/1
  MATLAB Function/7(Y7) -> Unit Delay4/1
  Data Type Conversion6/1 -> [X7]
  [X8] -> MATLAB Function/9(X8)
  [X7] -> MATLAB Function/8(X7)
  [X6] -> MATLAB Function/7(X6)
  [X5] -> MATLAB Function/6(X5)
  Data Type Conversion5/1 -> [X6]
  Data Type Conversion4/1 -> [X5]
  MATLAB Function/5(Y5) -> Unit Delay5/1
  MATLAB Function/6(Y6) -> Unit Delay6/1
  Unit Delay5/1 -> Data Type Conversion4/1
  Unit Delay6/1 -> Data Type Conversion5/1
  [X4] -> MATLAB Function/5(X4)
  [X3] -> MATLAB Function/4(X3)
  [X2] -> MATLAB Function/3(X2)
  Unit Delay3/1 -> Data Type Conversion3/1
  Unit Delay2/1 -> Data Type Conversion2/1
  Unit Delay1/1 -> Data Type Conversion1/1
  MATLAB Function/4(Y4) -> Unit Delay3/1
  MATLAB Function/3(Y3) -> Unit Delay2/1
  MATLAB Function/2(Y2) -> Unit Delay1/1
  C/1 -> MATLAB Function/1(C)
  MATLAB Function/1(S) -> Data Type Conversion9/1
  LFM1/1 -> MATLAB Function/2(Min)
  Data Type Conversion1/1 -> [X2]
  Data Type Conversion2/1 -> [X3]
  Data Type Conversion3/1 -> [X4]
  Data Type Conversion9/1 -> S/1

== system tpm/TPM/TPMS/TPMS/Learn/AutoLocation/IDIdentify/Subsystem7/Enabled Subsystem2 ==
  C : Inport
  LFM1 : Inport  Port=2
  Enable : EnablePort
  Data Type Conversion{1..8} (8 alike) : DataTypeConversion  OutDataTypeStr=int16
  Data Type Conversion9 : DataTypeConversion  OutDataTypeStr=uint8
  MATLAB Function : MATLAB Function  TreatAsAtomicUnit=on
  Unit Delay{1..8} (8 alike) : UnitDelay  SampleTime=-1  HasFrameUpgradeWarning=on
  S : Outport
  wires:
  Data Type Conversion3/1 -> [X4]
  Data Type Conversion2/1 -> [X3]
  Data Type Conversion1/1 -> [X2]
  LFM1/1 -> MATLAB Function/2(Min)
  MATLAB Function/1(S) -> Data Type Conversion9/1
  C/1 -> MATLAB Function/1(C)
  MATLAB Function/2(Y2) -> Unit Delay1/1
  MATLAB Function/3(Y3) -> Unit Delay2/1
  MATLAB Function/4(Y4) -> Unit Delay3/1
  Unit Delay1/1 -> Data Type Conversion1/1
  Unit Delay2/1 -> Data Type Conversion2/1
  Unit Delay3/1 -> Data Type Conversion3/1
  [X2] -> MATLAB Function/3(X2)
  [X3] -> MATLAB Function/4(X3)
  [X4] -> MATLAB Function/5(X4)
  Unit Delay6/1 -> Data Type Conversion5/1
  Unit Delay5/1 -> Data Type Conversion4/1
  MATLAB Function/6(Y6) -> Unit Delay6/1
  MATLAB Function/5(Y5) -> Unit Delay5/1
  Data Type Conversion4/1 -> [X5]
  Data Type Conversion5/1 -> [X6]
  [X5] -> MATLAB Function/6(X5)
  [X6] -> MATLAB Function/7(X6)
  [X7] -> MATLAB Function/8(X7)
  [X8] -> MATLAB Function/9(X8)
  Data Type Conversion6/1 -> [X7]
  MATLAB Function/7(Y7) -> Unit Delay4/1
  Unit Delay4/1 -> Data Type Conversion6/1
  Unit Delay7/1 -> Data Type Conversion7/1
  Data Type Conversion7/1 -> [X8]
  MATLAB Function/8(Y8) -> Unit Delay7/1
  MATLAB Function/9(Y9) -> Unit Delay8/1
  Data Type Conversion8/1 -> [X9]
  Unit Delay8/1 -> Data Type Conversion8/1
  [X9] -> MATLAB Function/10(X9)
  Data Type Conversion9/1 -> S/1

== system tpm/TPM/TPMS/TPMS/Learn/AutoLocation/IDIdentify/Subsystem7/Enabled Subsystem3 ==
  C : Inport
  LFM1 : Inport  Port=2
  Enable : EnablePort
  Data Type Conversion{1..8} (8 alike) : DataTypeConversion  OutDataTypeStr=int16
  Data Type Conversion9 : DataTypeConversion  OutDataTypeStr=uint8
  MATLAB Function : MATLAB Function  TreatAsAtomicUnit=on
  Unit Delay{1..8} (8 alike) : UnitDelay  SampleTime=-1  HasFrameUpgradeWarning=on
  S : Outport
  wires:
  [X9] -> MATLAB Function/10(X9)
  Unit Delay8/1 -> Data Type Conversion8/1
  Data Type Conversion8/1 -> [X9]
  MATLAB Function/9(Y9) -> Unit Delay8/1
  MATLAB Function/8(Y8) -> Unit Delay7/1
  Data Type Conversion7/1 -> [X8]
  Unit Delay7/1 -> Data Type Conversion7/1
  Unit Delay4/1 -> Data Type Conversion6/1
  MATLAB Function/7(Y7) -> Unit Delay4/1
  Data Type Conversion6/1 -> [X7]
  [X8] -> MATLAB Function/9(X8)
  [X7] -> MATLAB Function/8(X7)
  [X6] -> MATLAB Function/7(X6)
  [X5] -> MATLAB Function/6(X5)
  Data Type Conversion5/1 -> [X6]
  Data Type Conversion4/1 -> [X5]
  MATLAB Function/5(Y5) -> Unit Delay5/1
  MATLAB Function/6(Y6) -> Unit Delay6/1
  Unit Delay5/1 -> Data Type Conversion4/1
  Unit Delay6/1 -> Data Type Conversion5/1
  [X4] -> MATLAB Function/5(X4)
  [X3] -> MATLAB Function/4(X3)
  [X2] -> MATLAB Function/3(X2)
  Unit Delay3/1 -> Data Type Conversion3/1
  Unit Delay2/1 -> Data Type Conversion2/1
  Unit Delay1/1 -> Data Type Conversion1/1
  MATLAB Function/4(Y4) -> Unit Delay3/1
  MATLAB Function/3(Y3) -> Unit Delay2/1
  MATLAB Function/2(Y2) -> Unit Delay1/1
  C/1 -> MATLAB Function/1(C)
  MATLAB Function/1(S) -> Data Type Conversion9/1
  LFM1/1 -> MATLAB Function/2(Min)
  Data Type Conversion1/1 -> [X2]
  Data Type Conversion2/1 -> [X3]
  Data Type Conversion3/1 -> [X4]
  Data Type Conversion9/1 -> S/1

== system tpm/TPM/TPMS/TPMS/Learn/AutoLocation/IDIdentify/Subsystem7/Enabled Subsystem5 ==
  C : Inport
  LFM1 : Inport  Port=2
  Enable : EnablePort
  Data Type Conversion{1..8} (8 alike) : DataTypeConversion  OutDataTypeStr=int16
  Data Type Conversion9 : DataTypeConversion  OutDataTypeStr=uint8
  MATLAB Function : MATLAB Function  TreatAsAtomicUnit=on
  Unit Delay{1..8} (8 alike) : UnitDelay  SampleTime=-1  HasFrameUpgradeWarning=on
  S : Outport
  wires:
  Data Type Conversion3/1 -> [X4]
  Data Type Conversion2/1 -> [X3]
  Data Type Conversion1/1 -> [X2]
  LFM1/1 -> MATLAB Function/2(Min)
  MATLAB Function/1(S) -> Data Type Conversion9/1
  C/1 -> MATLAB Function/1(C)
  MATLAB Function/2(Y2) -> Unit Delay1/1
  MATLAB Function/3(Y3) -> Unit Delay2/1
  MATLAB Function/4(Y4) -> Unit Delay3/1
  Unit Delay1/1 -> Data Type Conversion1/1
  Unit Delay2/1 -> Data Type Conversion2/1
  Unit Delay3/1 -> Data Type Conversion3/1
  [X2] -> MATLAB Function/3(X2)
  [X3] -> MATLAB Function/4(X3)
  [X4] -> MATLAB Function/5(X4)
  Unit Delay6/1 -> Data Type Conversion5/1
  Unit Delay5/1 -> Data Type Conversion4/1
  MATLAB Function/6(Y6) -> Unit Delay6/1
  MATLAB Function/5(Y5) -> Unit Delay5/1
  Data Type Conversion4/1 -> [X5]
  Data Type Conversion5/1 -> [X6]
  [X5] -> MATLAB Function/6(X5)
  [X6] -> MATLAB Function/7(X6)
  [X7] -> MATLAB Function/8(X7)
  [X8] -> MATLAB Function/9(X8)
  Data Type Conversion6/1 -> [X7]
  MATLAB Function/7(Y7) -> Unit Delay4/1
  Unit Delay4/1 -> Data Type Conversion6/1
  Unit Delay7/1 -> Data Type Conversion7/1
  Data Type Conversion7/1 -> [X8]
  MATLAB Function/8(Y8) -> Unit Delay7/1
  MATLAB Function/9(Y9) -> Unit Delay8/1
  Data Type Conversion8/1 -> [X9]
  Unit Delay8/1 -> Data Type Conversion8/1
  [X9] -> MATLAB Function/10(X9)
  Data Type Conversion9/1 -> S/1

== system tpm/TPM/TPMS/TPMS/Learn/AutoLocation/WheelPosition/Subsystem/delay0 ==
  In1 : Inport
  Action Port : ActionPort
  Delay5 : Delay  DelayLength=0
  Out1 : Outport
  wires:
  In1/1 -> Delay5/1
  Delay5/1 -> Out1/1

== system tpm/TPM/TPMS/TPMS/Learn/AutoLocation/WheelPosition/Subsystem/delay1 ==
  In1 : Inport
  Action Port : ActionPort
  Delay5 : Delay  DelayLength=1
  Out1 : Outport
  wires:
  In1/1 -> Delay5/1
  Delay5/1 -> Out1/1

== system tpm/TPM/TPMS/TPMS/Learn/AutoLocation/WheelPosition/Subsystem/delay2 ==
  In1 : Inport
  Action Port : ActionPort
  Delay5 : Delay
  Out1 : Outport
  wires:
  In1/1 -> Delay5/1
  Delay5/1 -> Out1/1

== system tpm/TPM/TPMS/TPMS/Learn/AutoLocation/WheelPosition/Subsystem/delay3 ==
  In1 : Inport
  Action Port : ActionPort
  Delay5 : Delay  DelayLength=3
  Out1 : Outport
  wires:
  In1/1 -> Delay5/1
  Delay5/1 -> Out1/1

== system tpm/TPM/TPMS/TPMS/Learn/AutoLocation/WheelPosition/Subsystem/delay4 ==
  In1 : Inport
  Action Port : ActionPort
  Delay5 : Delay  DelayLength=4
  Out1 : Outport
  wires:
  Delay5/1 -> Out1/1
  In1/1 -> Delay5/1

== system tpm/TPM/TPMS/TPMS/Learn/AutoLocation/WheelPosition/Subsystem/delay5 ==
  In1 : Inport
  Action Port : ActionPort
  Delay5 : Delay  DelayLength=5
  Out1 : Outport
  wires:
  In1/1 -> Delay5/1
  Delay5/1 -> Out1/1

== system tpm/TPM/TPMS/TPMS/Learn/AutoLocation/WheelPosition/Subsystem/delay6 ==
  In1 : Inport
  Action Port : ActionPort
  Delay5 : Delay  DelayLength=6
  Out1 : Outport
  wires:
  Delay5/1 -> Out1/1
  In1/1 -> Delay5/1

== system tpm/TPM/TPMS/TPMS/Learn/AutoLocation/WheelPosition/Subsystem/delay7 ==
  In1 : Inport
  Action Port : ActionPort
  Delay5 : Delay  DelayLength=7
  Out1 : Outport
  wires:
  In1/1 -> Delay5/1
  Delay5/1 -> Out1/1

== system tpm/TPM/TPMS/TPMS/Learn/AutoLocation/WheelPosition/Subsystem/delay8 ==
  In1 : Inport
  Action Port : ActionPort
  Delay5 : Delay  DelayLength=8
  Out1 : Outport
  wires:
  Delay5/1 -> Out1/1
  In1/1 -> Delay5/1

== system tpm/TPM/TPMS/TPMS/Learn/AutoLocation/WheelPosition/Subsystem3/delay0 ==
  In1 : Inport
  Action Port : ActionPort
  Delay5 : Delay  DelayLength=0
  Out1 : Outport
  wires:
  Delay5/1 -> Out1/1
  In1/1 -> Delay5/1

== system tpm/TPM/TPMS/TPMS/Learn/AutoLocation/WheelPosition/Subsystem3/delay1 ==
  In1 : Inport
  Action Port : ActionPort
  Delay5 : Delay  DelayLength=1
  Out1 : Outport
  wires:
  Delay5/1 -> Out1/1
  In1/1 -> Delay5/1

== system tpm/TPM/TPMS/TPMS/Learn/AutoLocation/WheelPosition/Subsystem3/delay2 ==
  In1 : Inport
  Action Port : ActionPort  ActionPortLabel=elseif(u1 ==2)
  Delay5 : Delay
  Out1 : Outport
  wires:
  In1/1 -> Delay5/1
  Delay5/1 -> Out1/1

== system tpm/TPM/TPMS/TPMS/Learn/AutoLocation/WheelPosition/Subsystem3/delay3 ==
  In1 : Inport
  Action Port : ActionPort  ActionPortLabel=elseif(u1 ==3)
  Delay5 : Delay  DelayLength=3
  Out1 : Outport
  wires:
  Delay5/1 -> Out1/1
  In1/1 -> Delay5/1

== system tpm/TPM/TPMS/TPMS/Learn/AutoLocation/WheelPosition/Subsystem3/delay4 ==
  In1 : Inport
  Action Port : ActionPort
  Delay5 : Delay  DelayLength=4
  Out1 : Outport
  wires:
  In1/1 -> Delay5/1
  Delay5/1 -> Out1/1

== system tpm/TPM/TPMS/TPMS/Learn/AutoLocation/WheelPosition/Subsystem3/delay5 ==
  In1 : Inport
  Action Port : ActionPort
  Delay5 : Delay  DelayLength=5
  Out1 : Outport
  wires:
  Delay5/1 -> Out1/1
  In1/1 -> Delay5/1

== system tpm/TPM/TPMS/TPMS/Learn/AutoLocation/WheelPosition/Subsystem3/delay6 ==
  In1 : Inport
  Action Port : ActionPort
  Delay5 : Delay  DelayLength=6
  Out1 : Outport
  wires:
  In1/1 -> Delay5/1
  Delay5/1 -> Out1/1

== system tpm/TPM/TPMS/TPMS/Learn/AutoLocation/WheelPosition/Subsystem3/delay7 ==
  In1 : Inport
  Action Port : ActionPort
  Delay5 : Delay  DelayLength=7
  Out1 : Outport
  wires:
  Delay5/1 -> Out1/1
  In1/1 -> Delay5/1

== system tpm/TPM/TPMS/TPMS/Learn/AutoLocation/WheelPosition/Subsystem3/delay8 ==
  In1 : Inport
  Action Port : ActionPort
  Delay5 : Delay  DelayLength=8
  Out1 : Outport
  wires:
  In1/1 -> Delay5/1
  Delay5/1 -> Out1/1

== matlab function tpm/TPM/TPMS/TPMS/Learn/AutoLocation/IDIdentify/Subsystem7/Enabled Subsystem5/MATLAB Function ==
  data: C input; S output; Min input; X2 input; X3 input; X4 input; Y2 output; Y3 output; Y4 output; X5 input; X6 input; X7 input; X8 input; X9 input; Y5 output; Y6 output; Y7 output; Y8 output; Y9 output
function [S,Y2,Y3,Y4,Y5,Y6,Y7,Y8,Y9]   = fcn(C,Min,X2,X3,X4,X5,X6,X7,X8,X9)
Y=int16([X2 X3 X4 X5 X6 X7 X8 X9 Min]);
if (C<9)
    S=300;
else
    B=sort(Y);
    D=zeros(1,length(B));
    for i=1:1:length(D)
        if (i~=length(D))
            D(i)=B(i+1)-B(i);
        else
            if (B(length(D))-B(1)>B(1)+96-B(length(D)))
                D(length(D))=B(1)+96-B(length(D));
            else
                D(length(D))=B(length(D))-B(1);
            end
        end
    end

    [K,I]=sort(D);
    S=sum(K(1:7));
end
Y2=Y(2);
Y3=Y(3);
Y4=Y(4);
Y5=Y(5);
Y6=Y(6);
Y7=Y(7);
Y8=Y(8);
Y9=Y(9);

== stateflow chart tpm/TPM/TPMS/TPMS/Learn/AutoLocation/WheelPosition/Chart2 ==
  state Start
    state Forward
      en:
      a=(VTPM_RFWpos_raw+Delta);
      b=(VTPM_RFWpos_raw+Delta)/96;
      VTPM_RFWpos_raw=a-b*96;
    state Else
    state Backward
      en:
      a=(VTPM_RFWpos_raw+Delta);
      b=(VTPM_RFWpos_raw+Delta)/96;
      VTPM_RFWpos_raw=a-b*96;
    (default) -> (junction 54) : {VTPM_RFWpos_raw=0; Delta=0; PulseCountBuf=VINP_RFPulseCount_cnt;}
    Start -> (junction 54) : [hasChanged(VINP_RFPulseCount_cnt)]....
        | {Delta=VINP_RFPulseCount_cnt-PulseCountBuf;
        | PulseCountBuf=VINP_RFPulseCount_cnt;}
    (junction 54) -> (junction 47) [order 1] : [VPMM_PowerSta_enum!=ENUM_PWRSTASW_OFF&&....
        |  VPMM_PowerSta_enum!=ENUM_PWRSTASW_OFFCHVCHRG&&...
        |  VPMM_PowerSta_enum!=ENUM_PWRSTASW_OFFA&&....
        |  VPMM_PowerSta_enum!=ENUM_PWRSTASW_STANDBY&&....
        |  VINP_RFPulseCountV_flg==false]
    (junction 47) -> (junction 6) [order 1] : [VTPM_RFWhlRotDir_enum==1]
    (junction 6) -> Forward [order 1] : [Delta>0]
    (junction 54) -> Else [order 2]
    (junction 47) -> (junction 48) [order 2]
    (junction 6) -> (junction 10) [order 2] : [Delta<0]
    (junction 10) -> Forward : {Delta=Delta+256;}
    (junction 48) -> Else [order 2]
    (junction 48) -> (junction 14) [order 1] : [VTPM_RFWhlRotDir_enum==2]
    (junction 14) -> Backward [order 1] : [Delta>0]{Delta=-Delta+96;}
    (junction 14) -> (junction 16) [order 2] : [Delta<0]
    (junction 16) -> Backward : {Delta=-Delta+128;}
  data: VPMM_PowerSta_enum input; VINP_RFPulseCount_cnt input; VINP_RFPulseCountV_flg input; VTPM_RFWhlRotDir_enum input; VTPM_RFWpos_raw output int16; a local int16; b local int16; Delta local int16; PulseCountBuf local int16; ENUM_PWRSTASW_OFF parameter; ENUM_PWRSTASW_OFFA parameter; ENUM_PWRSTASW_OFFCHVCHRG parameter; ENUM_PWRSTASW_STANDBY parameter
